simulink model "lab10"  (R2019a)
settings: Solver=VariableStepAuto  StartTime=0.0  StopTime=10.0  RelTol=1e-3
model workspace (MAT data in the model file):
  V1 = 240
  V2 = 450
  V3 = 531
  k_01 = 0.231
  k_12 = 0.0438
  k_23 = 0.161
settings Model: OrderedModelArguments=off  Creator=sumli  LastModifiedBy=sumli

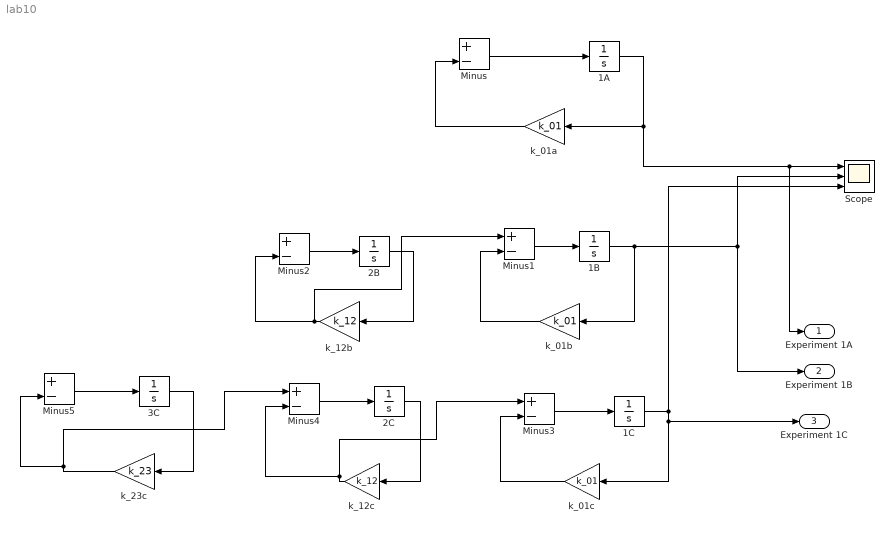
== system lab10 ==
  1A : Integrator  InitialCondition=300000/V1
  1B : Integrator
  1C : Integrator
  2B : Integrator  InitialCondition=300000/V2
  2C : Integrator
  3C : Integrator  InitialCondition=300000/V3
  Minus{,1..5} (6 alike) : Sum  Inputs=+-
  Scope : Scope  NumInputPorts=3
  k_01a : Gain  Gain=k_01
  k_01b : Gain  Gain=k_01
  k_01c : Gain  Gain=k_01
  k_12b : Gain  Gain=k_12
  k_12c : Gain  Gain=k_12
  k_23c : Gain  Gain=k_23
  Experiment 1A : Outport
  Experiment 1B : Outport  Port=2
  Experiment 1C : Outport  Port=3
  wires:
  Minus/1 -> 1A/1
  k_01a/1 -> Minus/2
  1A/1 -> Experiment 1A/1, Scope/1, k_01a/1
  1B/1 -> k_01b/1, Experiment 1B/1, Scope/2
  Minus1/1 -> 1B/1
  k_01b/1 -> Minus1/2
  2B/1 -> k_12b/1
  k_12b/1 -> Minus1/1, Minus2/2
  Minus2/1 -> 2B/1
  Minus3/1 -> 1C/1
  1C/1 -> Experiment 1C/1, k_01c/1, Scope/3
  k_01c/1 -> Minus3/2
  Minus4/1 -> 2C/1
  2C/1 -> k_12c/1
  k_12c/1 -> Minus3/1, Minus4/2
  3C/1 -> k_23c/1
  Minus5/1 -> 3C/1
  k_23c/1 -> Minus4/1, Minus5/2
